simulink model "sim_relay"  (R2025b)
settings: Solver=FixedStepAuto  StartTime=0.0  StopTime=Sim_time  FixedStep=dt  RelTol=1e-3
values from neighbouring files (symbols this model uses):
  J = 11.4    [relay_sim.m]
  Kd = 39.7    [relay_sim.m]
  Ki = 0.12    [relay_sim.m]
  Kp = 20    [relay_sim.m]
settings Model: Creator=3056709  LastModifiedBy=dharshini
settings DebuggingCC: UnconnectedInputMsg=warning  UnconnectedOutputMsg=warning  UnconnectedLineMsg=warning
settings ModelReferenceCC: EnableRefExpFcnMdlSchedulingChecks=on
settings RTWCC: GPUComputeCapability=3.5  DLArmComputeVersion=19.05

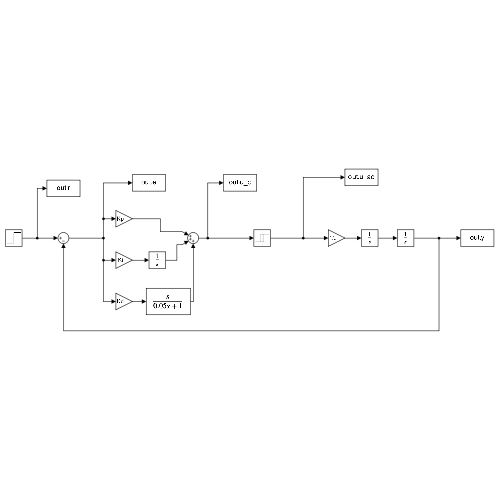
[thumbnail: Simulink's stored preview of the top-level diagram]
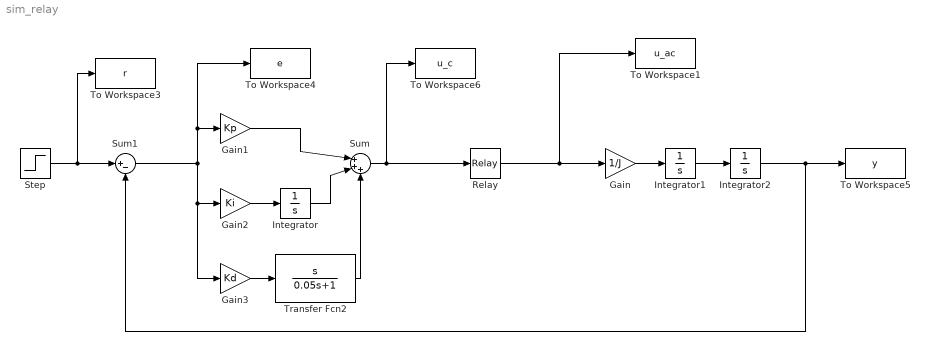
== system sim_relay ==
  Gain : Gain  Gain=1/J
  Gain1 : Gain  Gain=Kp
  Gain2 : Gain  Gain=Ki
  Gain3 : Gain  Gain=Kd
  Integrator : Integrator
  Integrator1 : Integrator
  Integrator2 : Integrator
  Relay : Relay  OnSwitchValue=0.7  OffSwitchValue=-0.7  OffOutputValue=-1
  Step : Step  Time=0  After=5  SampleTime=0
  Sum : Sum  Inputs=|+++
  Sum1 : Sum  Inputs=|+-
  To Workspace1 : ToWorkspace  VariableName=u_ac  SampleTime=-1
  To Workspace3 : ToWorkspace  VariableName=r  SampleTime=-1
  To Workspace4 : ToWorkspace  VariableName=e  SampleTime=-1
  To Workspace5 : ToWorkspace  VariableName=y  SampleTime=-1
  To Workspace6 : ToWorkspace  VariableName=u_c  SampleTime=-1
  Transfer Fcn2 : TransferFcn  Numerator=[1 0]  Denominator=[0.05 1]
  wires:
  Integrator2/1 -> To Workspace5/1, Sum1/2
  Gain1/1 -> Sum/1
  Gain2/1 -> Integrator/1
  Integrator/1 -> Sum/2
  Sum1/1 -> To Workspace4/1, Gain1/1, Gain3/1, Gain2/1
  Step/1 -> Sum1/1, To Workspace3/1
  Gain3/1 -> Transfer Fcn2/1
  Transfer Fcn2/1 -> Sum/3
  Gain/1 -> Integrator1/1
  Integrator1/1 -> Integrator2/1
  Sum/1 -> Relay/1, To Workspace6/1
  Relay/1 -> Gain/1, To Workspace1/1
